simulink model "Project2Week2Simulink"  (R2023b)
settings: Solver=VariableStepAuto  StartTime=0.0  StopTime=1200  RelTol=1e-3
values from neighbouring files (symbols this model uses):
  track_radius = 200    [init.m]
undefined symbols (not defined in the file or in its folder): carData
settings Model: Creator=joshc  LastModifiedBy=oscar

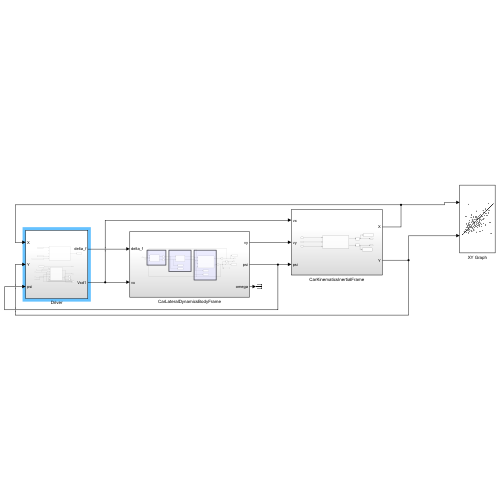
[thumbnail: Simulink's stored preview of the top-level diagram]
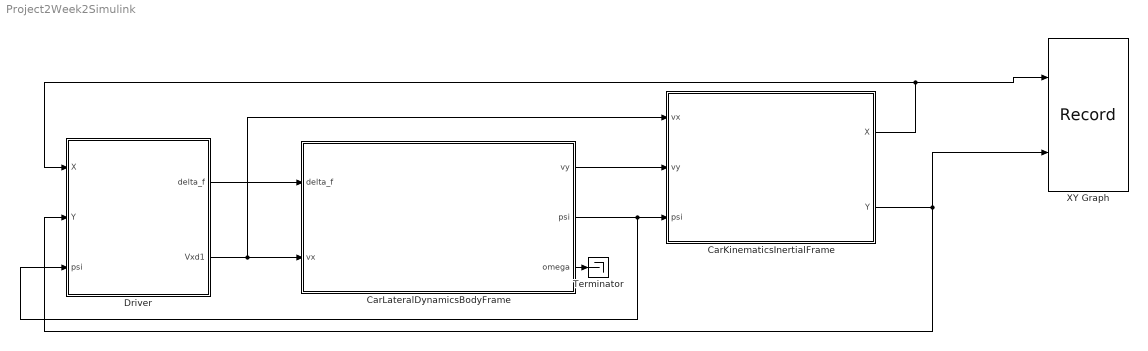
== system Project2Week2Simulink ==
  CarKinematicsInertialFrame : Subsystem
  CarLateralDynamicsBodyFrame : Subsystem
  Driver : Subsystem
  Terminator : Terminator
  XY Graph : Record  FileSettingsInternal="{\"entries\":[{\"content\":{\"excelSettings\":{\"content\":{},\"type\":\"Streamout.ExcelSettings\"}},\"type\":\"Streamout.FileSettingStorage\",\"uuid\":\"\"}],\"packageUris\":[\"http:\\/\\/schema.mathworks.com\\/mf0\\/streamout_blocks\\/R2020a\"],\"version\":\"1.0\"}"  Layout=[1 1]  SignalsInternal="{\"entries\":[{\"content\":{\"signals\":[{\"content\":{\"blockPath\":[],\"dimensions\":[1],\"domain\":\"\",\"lineColor\":\"#a2142f\",\"plots\":[1],\"port\":1,\"sid\":[\"\"],\"signalID\":6416,\"signalName\":\"CarKinematicsInertialFrame:1\"},\"type\":\"RecordBlkView.Signal\",\"uuid\":\"\"},{\"content\":{\"blockPath\":[],\"dimensions\":[1],\"domain\":\"\",\"lineColor\":\"#139fff\",\"plots\":[1],\"port\":2,\"sid\":[\"\"],\"signalID\":6420,\"signalName\":\"CarKinematicsInertialFrame:2\"},\"type\":\"RecordBlkView.Signal\",\"uuid\":\"\"}]},\"type\":\"RecordBlkView.InputSignals\",\"uuid\":\"\"}],\"packageUris\":[\"http:\\/\\/schema.mathworks.com\\/mf0\\/streamout_blocks\\/R2020a\"],\"version\":\"1.0\"}"  VisualizationBindings="{\"xyplotplugin\":{\"info\":[{\"series\":[{\"bindingParametersList\":[{\"parameter\":\"X-Axis\",\"signalID\":6416,\"signalName\":\"CarKinematicsInertialFrame:1\"},{\"parameter\":\"Y-Axis\",\"signalID\":6420,\"signalName\":\"CarKinematicsInertialFrame:2\"}],\"seriesID\":57789}],\"subplotID\":1}]}}"  CompatibilityTag=XY  st=-1
  wires:
  Driver/1(delta_f) -> CarLateralDynamicsBodyFrame/1(delta_f)
  CarKinematicsInertialFrame/1(X) -> Driver/1(X), XY Graph/1
  Driver/2(Vxd1) -> CarKinematicsInertialFrame/1(vx), CarLateralDynamicsBodyFrame/2(vx)
  CarLateralDynamicsBodyFrame/3(omega) -> Terminator/1
  CarLateralDynamicsBodyFrame/2(psi) -> Driver/3(psi), CarKinematicsInertialFrame/3(psi)
  CarLateralDynamicsBodyFrame/1(vy) -> CarKinematicsInertialFrame/2(vy)
  CarKinematicsInertialFrame/2(Y) -> Driver/2(Y), XY Graph/2

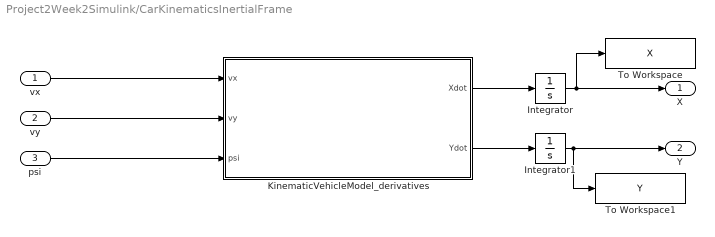
== system Project2Week2Simulink/CarKinematicsInertialFrame ==
  vx : Inport
  vy : Inport  Port=2
  psi : Inport  Port=3
  Integrator : Integrator  InitialCondition=carData.init.X0
  Integrator1 : Integrator  InitialCondition=carData.init.Y0
  KinematicVehicleModel_derivatives : MATLAB Function  TreatAsAtomicUnit=on  mask{obj=carData}
      mask prompts: obj "obj structure"
  To Workspace : ToWorkspace  VariableName=X  SaveFormat=Timeseries  SampleTime=-1
  To Workspace1 : ToWorkspace  VariableName=Y  SaveFormat=Timeseries  SampleTime=-1
  X : Outport
  Y : Outport  Port=2
  wires:
  KinematicVehicleModel_derivatives/1(Xdot) -> Integrator/1
  KinematicVehicleModel_derivatives/2(Ydot) -> Integrator1/1
  Integrator/1 -> To Workspace/1, X/1
  Integrator1/1 -> To Workspace1/1, Y/1
  vx/1 -> KinematicVehicleModel_derivatives/1(vx)
  vy/1 -> KinematicVehicleModel_derivatives/2(vy)
  psi/1 -> KinematicVehicleModel_derivatives/3(psi)

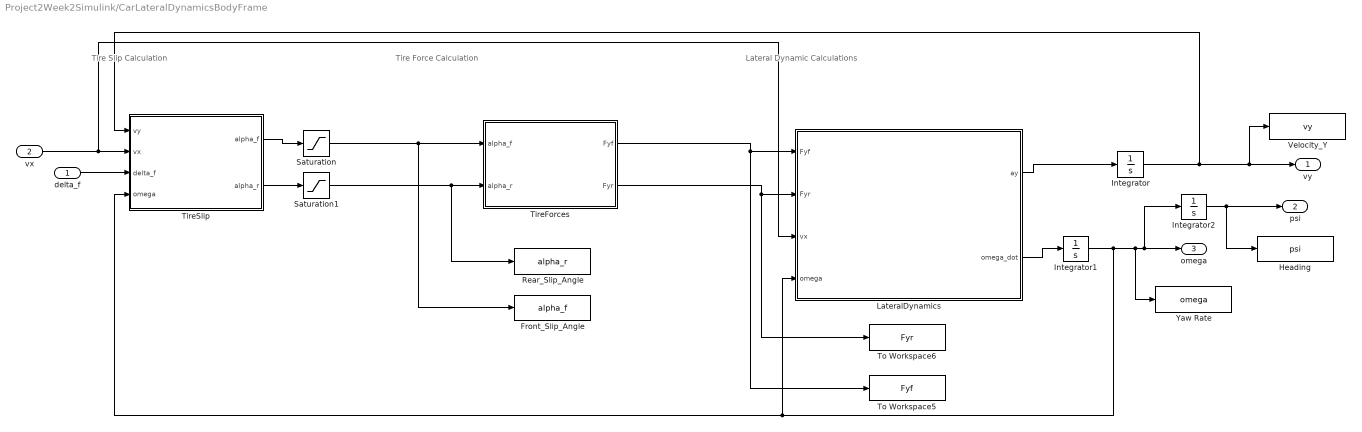
== system Project2Week2Simulink/CarLateralDynamicsBodyFrame ==
  note: Tire Slip Calculation
  note: Tire Force Calculation
  note: Lateral Dynamic Calculations
  delta_f : Inport
  vx : Inport  Port=2
  Front_Slip_Angle : ToWorkspace  VariableName=alpha_f  SaveFormat=Timeseries  SampleTime=-1
  Heading : ToWorkspace  VariableName=psi  SaveFormat=Timeseries  SampleTime=-1
  Integrator : Integrator  InitialCondition=carData.init.vy0
  Integrator1 : Integrator  InitialCondition=carData.init.omega0
  Integrator2 : Integrator  InitialCondition=carData.init.psi0  UpperSaturationLimit=2*pi  LowerSaturationLimit=0  WrappedStateUpperValue=pi*2  WrappedStateLowerValue=0
  LateralDynamics : MATLAB Function  TreatAsAtomicUnit=on  mask{obj=carData}
      mask prompts: obj "obj structure"
  Rear_Slip_Angle : ToWorkspace  VariableName=alpha_r  SaveFormat=Timeseries  SampleTime=-1
  Saturation : Saturate  UpperLimit=carData.maxAlpha  LowerLimit=-carData.maxAlpha
  Saturation1 : Saturate  UpperLimit=carData.maxAlpha  LowerLimit=-carData.maxAlpha
  TireForces : MATLAB Function  TreatAsAtomicUnit=on  mask{obj=carData}
      mask prompts: obj "obj structure"
  TireSlip : MATLAB Function  TreatAsAtomicUnit=on  mask{obj=carData}
      mask prompts: obj "obj structure"
  To Workspace5 : ToWorkspace  VariableName=Fyf  SaveFormat=Timeseries  SampleTime=-1
  To Workspace6 : ToWorkspace  VariableName=Fyr  SaveFormat=Timeseries  SampleTime=-1
  Velocity_Y : ToWorkspace  VariableName=vy  SaveFormat=Timeseries  SampleTime=-1
  Yaw Rate : ToWorkspace  VariableName=omega  SaveFormat=Timeseries  SampleTime=-1
  vy : Outport
  psi : Outport  Port=2
  omega : Outport  Port=3
  wires:
  LateralDynamics/1(ay) -> Integrator/1
  Integrator/1 -> vy/1, Velocity_Y/1, TireSlip/1(vy)
  LateralDynamics/2(omega_dot) -> Integrator1/1
  Integrator1/1 -> Integrator2/1, omega/1, Yaw Rate/1, LateralDynamics/4(omega), TireSlip/4(omega)
  TireSlip/1(alpha_f) -> Saturation/1
  TireSlip/2(alpha_r) -> Saturation1/1
  TireForces/1(Fyf) -> LateralDynamics/1(Fyf), To Workspace5/1
  TireForces/2(Fyr) -> LateralDynamics/2(Fyr), To Workspace6/1
  Saturation/1 -> TireForces/1(alpha_f), Front_Slip_Angle/1
  Saturation1/1 -> TireForces/2(alpha_r), Rear_Slip_Angle/1
  vx/1 -> TireSlip/2(vx), LateralDynamics/3(vx)
  delta_f/1 -> TireSlip/3(delta_f)
  Integrator2/1 -> Heading/1, psi/1

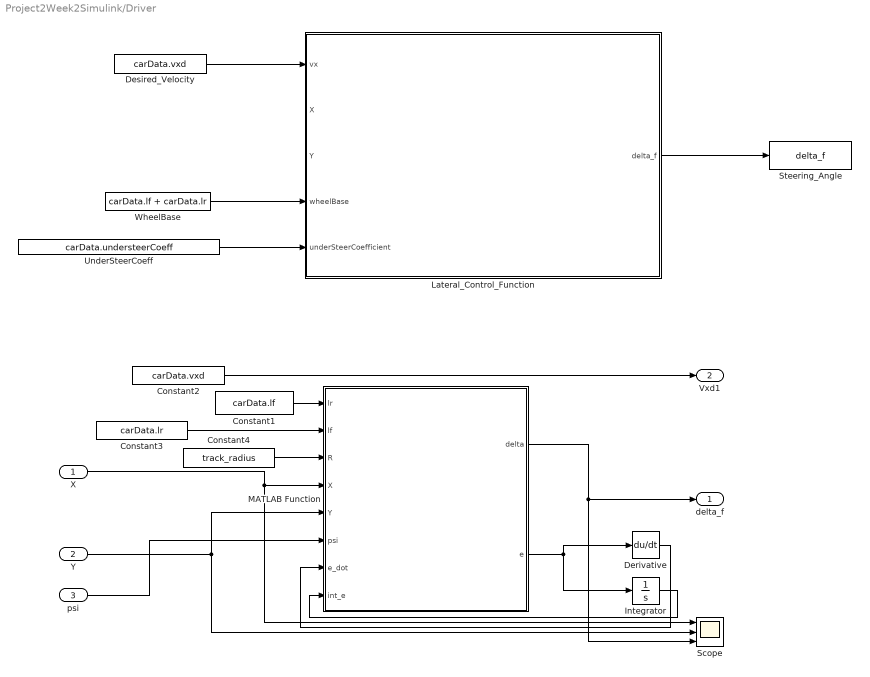
== system Project2Week2Simulink/Driver ==
  X : Inport
  Y : Inport  Port=2
  psi : Inport  Port=3
  Constant1 : Constant  Value=carData.lf
  Constant2 : Constant  Value=carData.vxd
  Constant3 : Constant  Value=carData.lr
  Constant4 : Constant  Value=track_radius
  Derivative : Derivative
  Desired_Velocity : Constant  Value=carData.vxd
  Integrator : Integrator  WrappedStateUpperValue=2*pi  WrappedStateLowerValue=0
  Lateral_Control_Function : MATLAB Function  TreatAsAtomicUnit=on
  MATLAB Function : MATLAB Function  TreatAsAtomicUnit=on
  Scope : Scope  NumInputPorts=3
  Steering_Angle : ToWorkspace  VariableName=delta_f  SaveFormat=Timeseries  SampleTime=-1
  UnderSteerCoeff : Constant  Value=carData.understeerCoeff
  WheelBase : Constant  Value=carData.lf + carData.lr
  delta_f : Outport
  Vxd1 : Outport  Port=2
  wires:
  Desired_Velocity/1 -> Lateral_Control_Function/1(vx)
  WheelBase/1 -> Lateral_Control_Function/4(wheelBase)
  Lateral_Control_Function/1(delta_f) -> Steering_Angle/1
  UnderSteerCoeff/1 -> Lateral_Control_Function/5(underSteerCoefficient)
  MATLAB Function/1(delta) -> delta_f/1, Scope/3
  Constant2/1 -> Vxd1/1
  X/1 -> MATLAB Function/4(X), Scope/1
  Y/1 -> Scope/2, MATLAB Function/5(Y)
  psi/1 -> MATLAB Function/6(psi)
  Constant1/1 -> MATLAB Function/1(lr)
  Constant3/1 -> MATLAB Function/2(lf)
  Constant4/1 -> MATLAB Function/3(R)
  MATLAB Function/2(e) -> Integrator/1, Derivative/1
  Integrator/1 -> MATLAB Function/8(int_e)
  Derivative/1 -> MATLAB Function/7(e_dot)

== matlab function Project2Week2Simulink/CarLateralDynamicsBodyFrame/LateralDynamics ==
  data: Fyf input; Fyr input size=1; vx input; omega input; ay output; obj parameter; omega_dot output
function [ay, omega_dot] = fcn(Fyf, Fyr, vx, omega, obj)

Fy = Fyf + Fyr;
ay = Fy / obj.Mass - omega * vx;
        
M  = Fyf * obj.lf - Fyr * obj.lr;        
omega_dot = M / obj.Inertia;        

end

== matlab function Project2Week2Simulink/Driver/Lateral_Control_Function ==
  data: vx input; delta_f output; X input; Y input; wheelBase input; underSteerCoefficient input
function delta_f   = latControl(vx,X,Y,wheelBase, underSteerCoefficient)

track_radius = 200;
track_length = 900;

track_seg1_x0 = 0;
track_seg1_y0 = 0;
track_seg1_x1 = track_length;
track_seg1_y1 = 0;
track_seg2_x0 = track_seg1_x1;
track_seg2_y0 = track_seg1_y1;
track_seg2_x1 = track_seg2_x0;
track_seg2_y1 = track_seg2_y0 + 2 * track_radius;
track_seg3_x0 = track_seg2_x1;
track_seg3_y0 = track_seg2_y1;
track_seg3_x1 = track_seg3_x0 - track_length;
track_seg3_y1 = track_seg3_y0;
track_seg4_x0 = track_seg3_x1;
track_seg4_y0 = track_seg3_y1;
track_seg4_x1 = track_seg1_x0;
track_seg4_y1 = track_seg1_y0;

if X > track_seg1_x0
    if X > track_seg1_x1
        segment = 2;
    else
        if Y > (track_seg2_y0 + track_seg2_y1)/2
            segment = 3;
        else
            segment = 1;
        end
    end
else
    segment = 4;
end



switch(segment)
    case 1
        delta_f = 0;
    case 2
        delta_f = - (wheelBase / track_radius + 1 * underSteerCoefficient * vx^2);
    case 3
        delta_f = 0;
    case 4
        delta_f = - (wheelBase / track_radius + 1 * underSteerCoefficient * vx^2);
    otherwise
        delta_f = 0;
end

== matlab function Project2Week2Simulink/CarKinematicsInertialFrame/KinematicVehicleModel_derivatives ==
  data: vx input; vy input; psi input size=1; Xdot output; Ydot output
function [Xdot, Ydot] = fcn(vx, vy, psi)
    temp = TF(psi) * [vx;vy] ; 
    Xdot = temp(1)-0.025;
    Ydot = temp(2);
    
end

function y = TF(psi)
    y = [cos(psi), -sin(psi); sin(psi), cos(psi)];
end

== matlab function Project2Week2Simulink/CarLateralDynamicsBodyFrame/TireSlip ==
  data: vy input size=1; vx input; delta_f input size=1; omega input; alpha_f output; obj parameter; alpha_r output
function [alpha_f, alpha_r] = fcn(vy,  vx, delta_f, omega, obj)


if abs(vx)> obj.vx_threshold1
      alpha_f = delta_f - (vy + omega * obj.lf) / vx;
      alpha_r = -(vy - omega * obj.lr) / vx;
else
      alpha_f = 0;
      alpha_r = 0;
end



end

== matlab function Project2Week2Simulink/CarLateralDynamicsBodyFrame/TireForces ==
  data: alpha_f input; alpha_r input; Fyf output; obj parameter; Fyr output
function [Fyf, Fyr] = fcn(alpha_f, alpha_r, obj)

Fyf = min(obj.Fyfmax,obj.Calpha_f * alpha_f);
Fyr = min(obj.Fyrmax, obj.Calpha_r * alpha_r);
end

== matlab function Project2Week2Simulink/Driver/MATLAB Function ==
  data: lr input; lf input; R input; X input; delta output; Y input; psi input; e_dot input; int_e input; e output
function [delta, e] = SimplestDriver(lr, lf, R, X, Y, psi, e_dot, int_e)

kp = 0;
kd = 0.05;
ki = 0;

psi_desired = (lr + lf) / R;
e = psi - psi_desired;

delta = 0;

if X >= 900
    if Y < 405
        PID = kp*e + kd*e_dot + ki*int_e;
        delta = PID + psi_desired;
    end
end

if X < 11
    if Y > 0
        PID = kp*e + kd*e_dot + ki*int_e;
        delta = (PID + psi_desired);
    end
end

if ((X > 0) && (X < 900)) && or((Y > 2),(Y < 2)) 
    delta = 0;
end
